simulink model "project"  (R2023b)
settings: Solver=FixedStepAuto  StartTime=0.0  StopTime=0.1  FixedStep=1e-6  RelTol=1e-3
values from neighbouring files (symbols this model uses):
  C_calculated = 0.000104    [project2.m]
  C_chosen = 0.0001    [project2.m]
  L_calculated = 0.006    [project2.m]
  L_chosen = 0.006    [project2.m]
  R = 2.4    [project2.m]
settings Model: Creator=trinc  LastModifiedBy=trinc

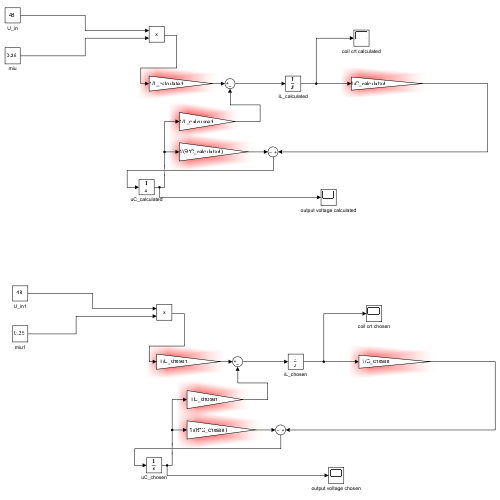
[thumbnail: Simulink's stored preview of the top-level diagram]
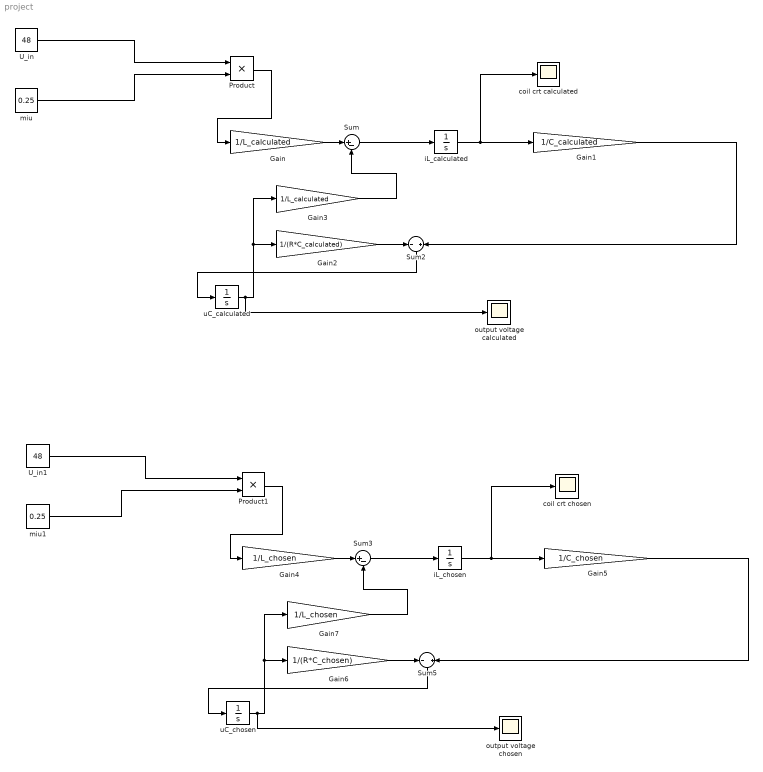
== system project ==
  Gain : Gain  Gain=1/L_calculated
  Gain1 : Gain  Gain=1/C_calculated
  Gain2 : Gain  Gain=1/(R*C_calculated)
  Gain3 : Gain  Gain=1/L_calculated
  Gain4 : Gain  Gain=1/L_chosen
  Gain5 : Gain  Gain=1/C_chosen
  Gain6 : Gain  Gain=1/(R*C_chosen)
  Gain7 : Gain  Gain=1/L_chosen
  Product : Product
  Product1 : Product
  Sum : Sum  Inputs=|+-
  Sum2 : Sum  Inputs=-||+
  Sum3 : Sum  Inputs=|+-
  Sum5 : Sum  Inputs=-||+
  U_in : Constant  Value=48
  U_in1 : Constant  Value=48
  coil crt calculated : Scope
  coil crt chosen : Scope
  iL_calculated : Integrator  InitialCondition=1
  iL_chosen : Integrator  InitialCondition=1
  miu : Constant  Value=0.25
  miu1 : Constant  Value=0.25
  output voltage calculated : Scope
  output voltage chosen : Scope
  uC_calculated : Integrator
  uC_chosen : Integrator
  wires:
  miu/1 -> Product/2
  Gain/1 -> Sum/1
  Sum/1 -> iL_calculated/1
  iL_calculated/1 -> coil crt calculated/1, Gain1/1
  Gain1/1 -> Sum2/2
  Gain2/1 -> Sum2/1
  Gain3/1 -> Sum/2
  U_in/1 -> Product/1
  Product/1 -> Gain/1
  Sum2/1 -> uC_calculated/1
  uC_calculated/1 -> Gain2/1, Gain3/1, output voltage calculated/1
  uC_chosen/1 -> Gain6/1, Gain7/1, output voltage chosen/1
  miu1/1 -> Product1/2
  iL_chosen/1 -> coil crt chosen/1, Gain5/1
  Gain5/1 -> Sum5/2
  Sum5/1 -> uC_chosen/1
  Gain4/1 -> Sum3/1
  U_in1/1 -> Product1/1
  Product1/1 -> Gain4/1
  Gain6/1 -> Sum5/1
  Gain7/1 -> Sum3/2
  Sum3/1 -> iL_chosen/1
